simulink model "replay"  (R2020a)
settings: Solver=VariableStepAuto  StartTime=0.0  StopTime=inf  RelTol=1e-3
model workspace (MAT data in the model file):
  Logfile_Data_Object = robotics.ros.BagSelection
  Logfile_Data_Object.FilePath = '/home/john/github/Thesis-/Control Algorithms/Navigation_Stack_2/Thesis Experiment Files/Outdoor-Waypoint-Navigation-Experiment/Outdoor-Waypoint-Navigation-Experiment-7/Outdoor-Waypoint-Navigation-Experiment-7.bag'
  Logfile_Data_Object.StartTime = 1662771107.21
  Logfile_Data_Object.EndTime = 1662771360.97
  Logfile_Data_Object.NumMessages = 71654
  Logfile_Data_Object.AvailableTopics = table
  Logfile_Data_Object.AvailableTopics.data{1} = [252; 252; 253; 4903; 2520; 32708; 2; 25371; 5186; 207]
  Logfile_Data_Object.AvailableTopics.data{2} = categorical
  Logfile_Data_Object.AvailableTopics.data{2}.categoryNames = {'geometry_msgs/Twist'; 'nav_msgs/OccupancyGrid'; 'nav_msgs/Odometry'; 'sensor_msgs/Imu'; 'sensor_msgs/LaserScan'; 'std_msgs/Float32'; 'std_msgs/Float32MultiArray'; 'tf2_msgs/TFMessage'}
  Logfile_Data_Object.AvailableTopics.data{2}.codes = [6; 6; 2; 3; 5; 8; 8; 4; 7; 1]
  Logfile_Data_Object.AvailableTopics.data{3}{1} = ''
  Logfile_Data_Object.AvailableTopics.data{3}{2} = ''
  Logfile_Data_Object.AvailableTopics.data{3}{3} = '  uint32 Seq
    |   Time Stamp
    |   char FrameId
    | nav_msgs/MapMetaData Info
    |   Time MapLoadTime
    |   single Resolution
    |   uint32 Width
    |   uint32 Height
    |   geometry_msgs/Pose Origin
    |     geometry_msgs/Point Position
    |       double X
    |       double Y
    |       double Z
    |     geometry_msgs/Quaternion Orientation
    |       double X
    |       double Y
    |       double Z
    |       double W
    | int8[] Data
    | '
  Logfile_Data_Object.AvailableTopics.data{3}{4} = '  uint32 Seq
    |   Time Stamp
    |   char FrameId
    | char ChildFrameId
    | geometry_msgs/PoseWithCovariance Pose
    |   geometry_msgs/Pose Pose
    |     geometry_msgs/Point Position
    |       double X
    |       double Y
    |       double Z
    |     geometry_msgs/Quaternion Orientation
    |       double X
    |       double Y
    |       double Z
    |       double W
    |   double[36] Covariance
    | geometry_msgs/TwistWithCovariance Twist
    |   geometry_msgs/Twist Twist
    |     geometry_msgs/Vector3 Linear
    |       double X
    |       double Y
    |       double Z
    |     geometry_msgs/Vector3 Angular
    |       double X
    |       double Y
    |       double Z
    |   double[36] Covariance
    | '
  Logfile_Data_Object.AvailableTopics.data{3}{5} = '  uint32 Seq
    |   Time Stamp
    |   char FrameId
    | single AngleMin
    | single AngleMax
    | single AngleIncrement
    | single TimeIncrement
    | single ScanTime
    | single RangeMin
    | single RangeMax
    | single[] Ranges
    | single[] Intensities
    | '
  Logfile_Data_Object.AvailableTopics.data{3}{6} = '  std_msgs/Header Header
    |     uint32 Seq
    |     Time Stamp
    |     char FrameId
    |   char ChildFrameId
    |   geometry_msgs/Transform Transform
    |     geometry_msgs/Vector3 Translation
    |       double X
    |       double Y
    |       double Z
    |     geometry_msgs/Quaternion Rotation
    |       double X
    |       double Y
    |       double Z
    |       double W
    | '
  Logfile_Data_Object.AvailableTopics.data{3}{7} = '  std_msgs/Header Header
    |     uint32 Seq
    |     Time Stamp
    |     char FrameId
    |   char ChildFrameId
    |   geometry_msgs/Transform Transform
    |     geometry_msgs/Vector3 Translation
    |       double X
    |       double Y
    |       double Z
    |     geometry_msgs/Quaternion Rotation
    |       double X
    |       double Y
    |       double Z
    |       double W
    | '
  Logfile_Data_Object.AvailableTopics.data{3}{8} = '  uint32 Seq
    |   Time Stamp
    |   char FrameId
    | geometry_msgs/Quaternion Orientation
    |   double X
    |   double Y
    |   double Z
    |   double W
    | double[9] OrientationCovariance
    | geometry_msgs/Vector3 AngularVelocity
    |   double X
    |   double Y
    |   double Z
    | double[9] AngularVelocityCovariance
    | geometry_msgs/Vector3 LinearAcceleration
    |   double X
    |   double Y
    |   double Z
    | double[9] LinearAccelerationCovariance
    | '
  Logfile_Data_Object.AvailableTopics.data{3}{9} = '  std_msgs/MultiArrayDimension[] Dim
    |     char Label
    |     uint32 Size
    |     uint32 Stride
    |   uint32 DataOffset
    | single[] Data
    | '
  Logfile_Data_Object.AvailableTopics.data{3}{10} = '  double X
    |   double Y
    |   double Z
    | geometry_msgs/Vector3 Angular
    |   double X
    |   double Y
    |   double Z
    | '
  Logfile_Data_Object.AvailableTopics.ndims = 2
  Logfile_Data_Object.AvailableTopics.nrows = 10
  Logfile_Data_Object.AvailableTopics.rownames = {'/amr/status/current'; '/amr/status/voltage'; '/slamware_ros_sdk_server_node/map'; '/slamware_ros_sdk_server_node/odom'; '/slamware_ros_sdk_server_node/scan'; '/tf'; '/tf_static'; '/tinkerforge_imu_ros/imu'; '/zlac8015d/encoder'; '/zlac8015d/rpm'}
  Logfile_Data_Object.AvailableTopics.nvars = 3
  Logfile_Data_Object.AvailableTopics.varnames = {'NumMessages', 'MessageType', 'MessageDefinition'}
  Logfile_Data_Object.AvailableTopics.props.useVariableNamesOriginal = 0
  Logfile_Data_Object.AvailableTopics.props.useDimensionNamesOriginal = 0
  Logfile_Data_Object.AvailableTopics.props.CustomProps = struct()
  Logfile_Data_Object.AvailableTopics.props.VariableCustomProps = struct()
  Logfile_Data_Object.AvailableTopics.props.versionSavedFrom = 4
  Logfile_Data_Object.AvailableTopics.props.minCompatibleVersion = 1
  Logfile_Data_Object.AvailableTopics.props.incompatibilityMsg = ''
  Logfile_Data_Object.AvailableTopics.props.VersionSavedFrom = 4
  Logfile_Data_Object.AvailableTopics.props.Description = ''
  Logfile_Data_Object.AvailableTopics.props.VariableNamesOriginal = {}
  Logfile_Data_Object.AvailableTopics.props.DimensionNames = {'Row', 'Variables'}
  Logfile_Data_Object.AvailableTopics.props.DimensionNamesOriginal = {}
  Logfile_Data_Object.AvailableTopics.props.UserData = []
  Logfile_Data_Object.AvailableTopics.props.VariableDescriptions = {}
  Logfile_Data_Object.AvailableTopics.props.VariableUnits = {}
  Logfile_Data_Object.AvailableTopics.props.VariableContinuity = {}
  Logfile_Data_Object.AvailableFrames = {'base_link'; 'base_link_z'; 'imu_link'; 'laser'; 'map'; 'odom'; 'odom_z'; 'remapped_laser'; 'slamware_map'; 'zed2_baro_link'; 'zed2_base_link'; 'zed2_camera_center'; 'zed2_imu_link'; 'zed2_left_camera_frame'; 'zed2_left_camera_optical_frame'; 'zed2_mag_link'; 'zed2_right_camera_frame'; 'zed2_right_camera_optical_frame'; 'zed2_temp_left_link'; 'zed2_temp_right_link'}
  Logfile_Data_Object.MessageList = table
  Logfile_Data_Object.MessageList.data{1} = [1662771107.21 1662771107.21 1662771107.21 1662771107.21 1662771107.21 1662771107.21 1662771107.21 1662771107.21 1662771107.21 1662771107.21 1662771107.21 1662771107.21 ... (71654 elements, 71654x1)]
  Logfile_Data_Object.MessageList.data{2} = categorical
  Logfile_Data_Object.MessageList.data{2}.categoryNames = {'/amr/status/current'; '/amr/status/voltage'; '/slamware_ros_sdk_server_node/map'; '/slamware_ros_sdk_server_node/odom'; '/slamware_ros_sdk_server_node/scan'; '/tf'; '/tf_static'; '/tinkerforge_imu_ros/imu'; '/zlac8015d/encoder'; '/zlac8015d/rpm'}
  Logfile_Data_Object.MessageList.data{2}.codes = [6 7 6 6 6 6 6 6 6 6 6 6 ... (71654 elements, 71654x1)]
  Logfile_Data_Object.MessageList.data{3} = categorical
  Logfile_Data_Object.MessageList.data{3}.categoryNames = {'std_msgs/Float32'; 'nav_msgs/OccupancyGrid'; 'nav_msgs/Odometry'; 'sensor_msgs/LaserScan'; 'tf2_msgs/TFMessage'; 'sensor_msgs/Imu'; 'std_msgs/Float32MultiArray'; 'geometry_msgs/Twist'}
  Logfile_Data_Object.MessageList.data{3}.codes = [5 5 5 5 5 5 5 5 5 5 5 5 ... (71654 elements, 71654x1)]
  Logfile_Data_Object.MessageList.data{4} = [6407 8809 10010 10163 10306 10450 10592 10745 10892 11035 11179 11321 ... (71654 elements, 71654x1)]
  Logfile_Data_Object.MessageList.ndims = 2
  Logfile_Data_Object.MessageList.nrows = 71654
  Logfile_Data_Object.MessageList.nvars = 4
  Logfile_Data_Object.MessageList.varnames = {'Time', 'Topic', 'MessageType', 'FileOffset'}
  Logfile_Data_Object.MessageList.props.useVariableNamesOriginal = 0
  Logfile_Data_Object.MessageList.props.useDimensionNamesOriginal = 0
  Logfile_Data_Object.MessageList.props.CustomProps = struct()
  Logfile_Data_Object.MessageList.props.VariableCustomProps = struct()
  Logfile_Data_Object.MessageList.props.versionSavedFrom = 4
  Logfile_Data_Object.MessageList.props.minCompatibleVersion = 1
  Logfile_Data_Object.MessageList.props.incompatibilityMsg = ''
  Logfile_Data_Object.MessageList.props.VersionSavedFrom = 4
  Logfile_Data_Object.MessageList.props.Description = ''
  Logfile_Data_Object.MessageList.props.VariableNamesOriginal = {}
  Logfile_Data_Object.MessageList.props.DimensionNames = {'Row', 'Variables'}
  Logfile_Data_Object.MessageList.props.DimensionNamesOriginal = {}
  Logfile_Data_Object.MessageList.props.UserData = []
  Logfile_Data_Object.MessageList.props.VariableDescriptions = {}
  Logfile_Data_Object.MessageList.props.VariableUnits = {}
  Logfile_Data_Object.MessageList.props.VariableContinuity = {}
  Logfile_Data_Object.TopicTypeMap = containers.Map
  Logfile_Data_Object.TopicTypeMap.serialization.keys = {'/amr/status/current', '/amr/status/voltage', '/slamware_ros_sdk_server_node/map', '/slamware_ros_sdk_server_node/odom', '/slamware_ros_sdk_server_node/scan', '/tf', '/tf_static', '/tinkerforge_imu_ros/imu', '/zlac8015d/encoder', '/zlac8015d/rpm'}
  Logfile_Data_Object.TopicTypeMap.serialization.values = {'std_msgs/Float32', 'std_msgs/Float32', 'nav_msgs/OccupancyGrid', 'nav_msgs/Odometry', 'sensor_msgs/LaserScan', 'tf2_msgs/TFMessage', 'tf2_msgs/TFMessage', 'sensor_msgs/Imu', 'std_msgs/Float32MultiArray', 'geometry_msgs/Twist'}
  Logfile_Data_Object.TopicTypeMap.serialization.uniformity = 1
  Logfile_Data_Object.TopicTypeMap.serialization.keyType = 'char'
  Logfile_Data_Object.TopicTypeMap.serialization.valueType = 'char'
  Logfile_Data_Object.TopicDefinitionMap = containers.Map
  Logfile_Data_Object.TopicDefinitionMap.serialization.keys = {'/amr/status/current', '/amr/status/voltage', '/slamware_ros_sdk_server_node/map', '/slamware_ros_sdk_server_node/odom', '/slamware_ros_sdk_server_node/scan', '/tf', '/tf_static', '/tinkerforge_imu_ros/imu', '/zlac8015d/encoder', '/zlac8015d/rpm'}
  Logfile_Data_Object.TopicDefinitionMap.serialization.values{1} = ''
  Logfile_Data_Object.TopicDefinitionMap.serialization.values{2} = ''
  Logfile_Data_Object.TopicDefinitionMap.serialization.values{3} = '  uint32 Seq
    |   Time Stamp
    |   char FrameId
    | nav_msgs/MapMetaData Info
    |   Time MapLoadTime
    |   single Resolution
    |   uint32 Width
    |   uint32 Height
    |   geometry_msgs/Pose Origin
    |     geometry_msgs/Point Position
    |       double X
    |       double Y
    |       double Z
    |     geometry_msgs/Quaternion Orientation
    |       double X
    |       double Y
    |       double Z
    |       double W
    | int8[] Data
    | '
  Logfile_Data_Object.TopicDefinitionMap.serialization.values{4} = '  uint32 Seq
    |   Time Stamp
    |   char FrameId
    | char ChildFrameId
    | geometry_msgs/PoseWithCovariance Pose
    |   geometry_msgs/Pose Pose
    |     geometry_msgs/Point Position
    |       double X
    |       double Y
    |       double Z
    |     geometry_msgs/Quaternion Orientation
    |       double X
    |       double Y
    |       double Z
    |       double W
    |   double[36] Covariance
    | geometry_msgs/TwistWithCovariance Twist
    |   geometry_msgs/Twist Twist
    |     geometry_msgs/Vector3 Linear
    |       double X
    |       double Y
    |       double Z
    |     geometry_msgs/Vector3 Angular
    |       double X
    |       double Y
    |       double Z
    |   double[36] Covariance
    | '
  Logfile_Data_Object.TopicDefinitionMap.serialization.values{5} = '  uint32 Seq
    |   Time Stamp
    |   char FrameId
    | single AngleMin
    | single AngleMax
    | single AngleIncrement
    | single TimeIncrement
    | single ScanTime
    | single RangeMin
    | single RangeMax
    | single[] Ranges
    | single[] Intensities
    | '
  Logfile_Data_Object.TopicDefinitionMap.serialization.values{6} = '  std_msgs/Header Header
    |     uint32 Seq
    |     Time Stamp
    |     char FrameId
    |   char ChildFrameId
    |   geometry_msgs/Transform Transform
    |     geometry_msgs/Vector3 Translation
    |       double X
    |       double Y
    |       double Z
    |     geometry_msgs/Quaternion Rotation
    |       double X
    |       double Y
    |       double Z
    |       double W
    | '
  Logfile_Data_Object.TopicDefinitionMap.serialization.values{7} = '  std_msgs/Header Header
    |     uint32 Seq
    |     Time Stamp
    |     char FrameId
    |   char ChildFrameId
    |   geometry_msgs/Transform Transform
    |     geometry_msgs/Vector3 Translation
    |       double X
    |       double Y
    |       double Z
    |     geometry_msgs/Quaternion Rotation
    |       double X
    |       double Y
    |       double Z
    |       double W
    | '
  Logfile_Data_Object.TopicDefinitionMap.serialization.values{8} = '  uint32 Seq
    |   Time Stamp
    |   char FrameId
    | geometry_msgs/Quaternion Orientation
    |   double X
    |   double Y
    |   double Z
    |   double W
    | double[9] OrientationCovariance
    | geometry_msgs/Vector3 AngularVelocity
    |   double X
    |   double Y
    |   double Z
    | double[9] AngularVelocityCovariance
    | geometry_msgs/Vector3 LinearAcceleration
    |   double X
    |   double Y
    |   double Z
    | double[9] LinearAccelerationCovariance
    | '
  Logfile_Data_Object.TopicDefinitionMap.serialization.values{9} = '  std_msgs/MultiArrayDimension[] Dim
    |     char Label
    |     uint32 Size
    |     uint32 Stride
    |   uint32 DataOffset
    | single[] Data
    | '
  Logfile_Data_Object.TopicDefinitionMap.serialization.values{10} = '  double X
    |   double Y
    |   double Z
    | geometry_msgs/Vector3 Angular
    |   double X
    |   double Y
    |   double Z
    | '
  Logfile_Data_Object.TopicDefinitionMap.serialization.uniformity = 1
  Logfile_Data_Object.TopicDefinitionMap.serialization.keyType = 'char'
  Logfile_Data_Object.TopicDefinitionMap.serialization.valueType = 'char'
  Logfile_Data_Object.Parser = robotics.ros.internal.tf.TransformationTreeParser
  Logfile_Path = '/home/john/github/Thesis-/Control Algorithms/Navigation_Stack_2/Thesis Experiment Files/Outdoor-Waypoint-Navigation-Experiment/Outdoor-Waypoint-Navigation-Experiment-7/Outdoor-Waypoint-Navigation-Experiment-7.bag'
  Logfile_Playback_Duration = nan
  Logfile_Playback_Offset = nan
values from neighbouring files (symbols this model uses):
  W2ORTransform = [cos(W2ORtheta), -sin(W2ORtheta), W2ORx ... (first row only)    [startup.m]
libraries: robotlib x2
settings Model: EnablePacing=on  Creator=john  LastModifiedBy=john

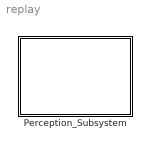
== system replay ==
  Perception_Subsystem : Subsystem

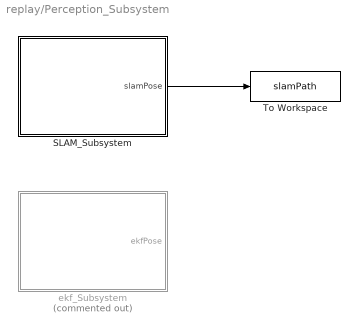
== system replay/Perception_Subsystem ==
  SLAM_Subsystem : Subsystem
  To Workspace : ToWorkspace  VariableName=slamPath  SaveFormat=Timeseries  SampleTime=-1
  ekf_Subsystem : Subsystem  Commented=on
  wires:
  SLAM_Subsystem/1(slamPose) -> To Workspace/1

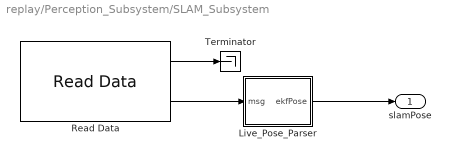
== system replay/Perception_Subsystem/SLAM_Subsystem ==
  Live_Pose_Parser : Subsystem
  Read Data : robotlib/Read Data  topic=/slamware_ros_sdk_server_node/odom  sampleTime=-1  logfileType=rosbag  modelName=replay  msgType=nav_msgs/Odometry
      settings: SourceProductBaseCode=RR
  Terminator : Terminator
  slamPose : Outport
  wires:
  Live_Pose_Parser/1(ekfPose) -> slamPose/1
  Read Data/1 -> Terminator/1
  Read Data/2 -> Live_Pose_Parser/1(msg)

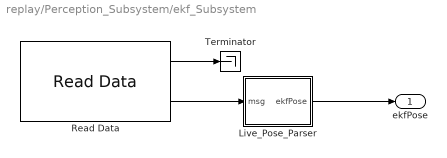
== system replay/Perception_Subsystem/ekf_Subsystem ==
  Live_Pose_Parser : Subsystem
  Read Data : robotlib/Read Data  topic=/my_topic  sampleTime=-1  logfileType=rosbag  modelName=replay
      settings: SourceProductBaseCode=RR
  Terminator : Terminator
  ekfPose : Outport
  wires:
  Read Data/2 -> Live_Pose_Parser/1(msg)
  Read Data/1 -> Terminator/1
  Live_Pose_Parser/1(ekfPose) -> ekfPose/1

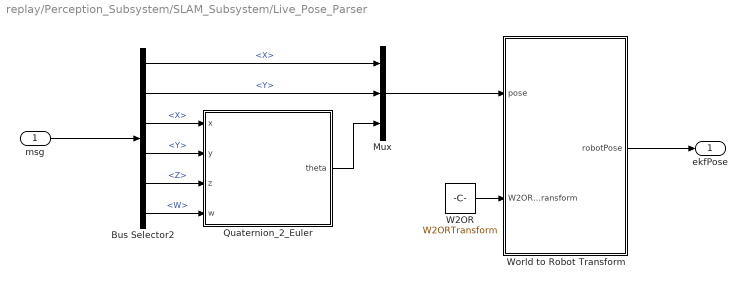
== system replay/Perception_Subsystem/SLAM_Subsystem/Live_Pose_Parser ==
  msg : Inport
  Bus Selector2 : BusSelector  OutputSignals=Pose.Pose.Position.X,Pose.Pose.Position.Y,Pose.Pose.Orientation.X,Pose.Pose.Orientation.Y,Pose.Pose.Orientation.Z,Pose.Pose.Orientation.W
  Mux : Mux  Inputs=3
  Quaternion_2_Euler : MATLAB Function  TreatAsAtomicUnit=on
  W2OR : Constant  Value=W2ORTransform
  World to Robot Transform : MATLAB Function  TreatAsAtomicUnit=on
  ekfPose : Outport
  wires:
  msg/1 -> Bus Selector2/1
  Bus Selector2/1 -> Mux/1  "<X>"
  Bus Selector2/2 -> Mux/2  "<Y>"
  Bus Selector2/3 -> Quaternion_2_Euler/1(x)  "<X>"
  Bus Selector2/4 -> Quaternion_2_Euler/2(y)  "<Y>"
  Bus Selector2/5 -> Quaternion_2_Euler/3(z)  "<Z>"
  Bus Selector2/6 -> Quaternion_2_Euler/4(w)  "<W>"
  Quaternion_2_Euler/1(theta) -> Mux/3
  Mux/1 -> World to Robot Transform/1(pose)
  World to Robot Transform/1(robotPose) -> ekfPose/1
  W2OR/1 -> World to Robot Transform/2(W2ORTransform)

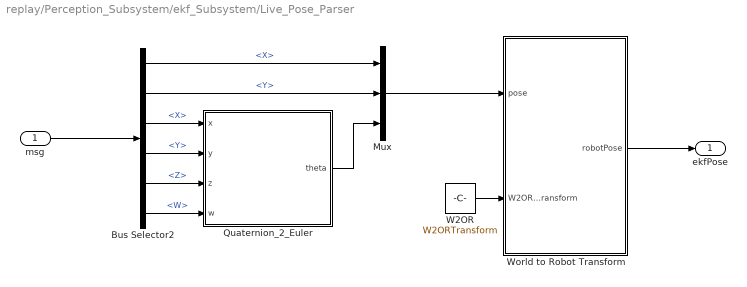
== system replay/Perception_Subsystem/ekf_Subsystem/Live_Pose_Parser ==
  msg : Inport
  Bus Selector2 : BusSelector  OutputSignals=Pose.Pose.Position.X,Pose.Pose.Position.Y,Pose.Pose.Orientation.X,Pose.Pose.Orientation.Y,Pose.Pose.Orientation.Z,Pose.Pose.Orientation.W
  Mux : Mux  Inputs=3
  Quaternion_2_Euler : MATLAB Function  TreatAsAtomicUnit=on
  W2OR : Constant  Value=W2ORTransform
  World to Robot Transform : MATLAB Function  TreatAsAtomicUnit=on
  ekfPose : Outport
  wires:
  msg/1 -> Bus Selector2/1
  Bus Selector2/1 -> Mux/1  "<X>"
  Bus Selector2/2 -> Mux/2  "<Y>"
  Bus Selector2/3 -> Quaternion_2_Euler/1(x)  "<X>"
  Bus Selector2/4 -> Quaternion_2_Euler/2(y)  "<Y>"
  Bus Selector2/5 -> Quaternion_2_Euler/3(z)  "<Z>"
  Bus Selector2/6 -> Quaternion_2_Euler/4(w)  "<W>"
  Quaternion_2_Euler/1(theta) -> Mux/3
  Mux/1 -> World to Robot Transform/1(pose)
  World to Robot Transform/1(robotPose) -> ekfPose/1
  W2OR/1 -> World to Robot Transform/2(W2ORTransform)

== matlab function replay/Perception_Subsystem/SLAM_Subsystem/Live_Pose_Parser/Quaternion_2_Euler ==
  data: x input; theta output; y input; z input; w input
function theta = fcn(x, y, z, w)

    euler = quat2eul([x, y, z, w]); 
    
    if sum(isnan(euler)) == 3
        
        euler = ([pi, 0, 0]);
        
    end 
    
theta = euler(1,3);

== matlab function replay/Perception_Subsystem/SLAM_Subsystem/Live_Pose_Parser/World to Robot Transform ==
  data: pose input; robotPose output; W2ORTransform input
function robotPose = fcn(pose, W2ORTransform)
    
    % Robot to Odom   
    OR2RTransform = [cos(pose(3,1)), -sin(pose(3,1)), pose(1,1);
                    sin(pose(3,1)), cos(pose(3,1)), pose(2,1);
                    0,              0,              1];

    % Calculate World to Robot
    W2RTransform = W2ORTransform*OR2RTransform; 
    

    % Extract relevant information
robotPose = [W2RTransform(1,3); W2RTransform(2,3); acos(W2RTransform(1,1))];

== matlab function replay/Perception_Subsystem/ekf_Subsystem/Live_Pose_Parser/Quaternion_2_Euler ==
  data: x input; theta output; y input; z input; w input
function theta = fcn(x, y, z, w)

    euler = quat2eul([x, y, z, w]); 
    
    if sum(isnan(euler)) == 3
        
        euler = ([pi, 0, 0]);
        
    end 
    
theta = euler(1,3);

== matlab function replay/Perception_Subsystem/ekf_Subsystem/Live_Pose_Parser/World to Robot Transform ==
  data: pose input; robotPose output; W2ORTransform input
function robotPose = fcn(pose, W2ORTransform)
    
    % Robot to Odom   
    OR2RTransform = [cos(pose(3,1)), -sin(pose(3,1)), pose(1,1);
                    sin(pose(3,1)), cos(pose(3,1)), pose(2,1);
                    0,              0,              1];

    % Calculate World to Robot
    W2RTransform = W2ORTransform*OR2RTransform; 
    

    % Extract relevant information
robotPose = [W2RTransform(1,3); W2RTransform(2,3); acos(W2RTransform(1,1))];
